simulink model "f_cd_reorder"  (R2018a)
settings: Solver=VariableStepAuto  StartTime=0.0  StopTime=200000  RelTol=1e-3
libraries: xbsIndex_r4 x1711, casper_library_misc x12, xps_library x2, simulink x1
(part 9 of 9)

== system f_cd_reorder/hmc_cd_reorder/reord/Subsystem/write_counter0 ==
  note: if there is a value missing we want to
      | increase by 1, if an enable we want to
      | increment by 2. If both then 3
  rst : Inport
  en : Inport  Port=2
  missing : Inport  Port=3
  AddSub2 : xbsIndex_r4/AddSub  mode=Addition  use_carryin=off  use_carryout=off  en=off  latency=0  precision=User Defined  arith_type=Unsigned  n_bits=n_bits_buffer  bin_pt=0  quantization=Truncate  overflow=Wrap  use_behavioral_HDL=on  hw_selection=Fabric  pipelined=off  dbl_ovrd=off  block_type=addsub
  Concat : xbsIndex_r4/Concat  num_inputs=2  dbl_ovrd=off  block_type=concat
  Constant : xbsIndex_r4/Constant  const=1  gui_display_data_type=Fixed-point  arith_type=Unsigned  n_bits=2  bin_pt=0  preci_type=Single  exp_width=8  frac_width=24  explicit_period=on  period=1  equ=P=C  opselect=C  inp2=PCIN>>17  opr=+  inp1=P  carry=CIN  dbl_ovrd=off  block_type=constant
  Constant1 : xbsIndex_r4/Constant  const=3  gui_display_data_type=Fixed-point  arith_type=Unsigned  n_bits=2  bin_pt=0  preci_type=Single  exp_width=8  frac_width=24  explicit_period=on  period=1  equ=P=C  opselect=C  inp2=PCIN>>17  opr=+  inp1=P  carry=CIN  dbl_ovrd=off  block_type=constant
  Constant2 : xbsIndex_r4/Constant  const=2  gui_display_data_type=Fixed-point  arith_type=Unsigned  n_bits=2  bin_pt=0  preci_type=Single  exp_width=8  frac_width=24  explicit_period=on  period=1  equ=P=C  opselect=C  inp2=PCIN>>17  opr=+  inp1=P  carry=CIN  dbl_ovrd=off  block_type=constant
  Constant3 : xbsIndex_r4/Constant  const=0  gui_display_data_type=Fixed-point  arith_type=Unsigned  n_bits=2  bin_pt=0  preci_type=Single  exp_width=8  frac_width=24  explicit_period=on  period=1  equ=P=C  opselect=C  inp2=PCIN>>17  opr=+  inp1=P  carry=CIN  dbl_ovrd=off  block_type=constant
  Delay13 : xbsIndex_r4/Delay  rst=off  infoeditControl=Selection of Reset will increase slice count due to use of real FFs and instead of SRLs  en=off  latency=1  reg_retiming=on  dbl_ovrd=off  block_type=delay
  Delay2 : xbsIndex_r4/Delay  rst=off  infoeditControl=Selection of Reset will increase slice count due to use of real FFs and instead of SRLs  en=off  latency=2  reg_retiming=on  dbl_ovrd=off  block_type=delay
  Delay3 : xbsIndex_r4/Delay  rst=off  infoeditControl=Selection of Reset will increase slice count due to use of real FFs and instead of SRLs  en=off  latency=2  reg_retiming=on  dbl_ovrd=off  block_type=delay
  Delay4 : xbsIndex_r4/Delay  rst=off  infoeditControl=Selection of Reset will increase slice count due to use of real FFs and instead of SRLs  en=off  latency=2  reg_retiming=on  dbl_ovrd=off  block_type=delay
  Gateway Out{,1..5} (6 alike) : xbsIndex_r4/Gateway Out  inherit_from_input=off  hdl_port=off  rows=1  columns=1  UseAsDAC=off  DACChannel='1'  interface=None  automatic_assignment=on  address_offset=hex2dec('00')  intf_name=''  intf_description=''  timing_constraint=None  locs_specified=off  LOCs={}  io_standard={}  block_type=gatewayout
  Logical8 : xbsIndex_r4/Logical  logical_function=OR  inputs=2  en=off  latency=1  precision=Full  arith_type=Unsigned  n_bits=16  bin_pt=0  align_bp=on  dbl_ovrd=off  block_type=logical
  Mux1 : xbsIndex_r4/Mux  inputs=4  en=off  latency=1  precision=Full  arith_type=Unsigned  n_bits=16  bin_pt=14  quantization=Truncate  overflow=Wrap  dbl_ovrd=off  block_type=mux
  Register : xbsIndex_r4/Register  init=0  rst=on  en=on  dbl_ovrd=off  block_type=register
  Scope : Scope  NumInputPorts=6
  count : Outport
  wires:
  en/1 -> Delay3/1
  AddSub2/1 -> Register/1, Gateway Out4/1
  rst/1 -> Delay4/1
  Delay13/1 -> Register/2
  missing/1 -> Delay2/1
  Logical8/1 -> Register/3
  Mux1/1 -> Gateway Out3/1, AddSub2/1
  Concat/1 -> Mux1/1
  Gateway Out/1 -> Scope/1
  Gateway Out1/1 -> Scope/2
  Gateway Out2/1 -> Scope/3
  Gateway Out3/1 -> Scope/4
  Gateway Out4/1 -> Scope/5
  Gateway Out5/1 -> Scope/6
  Constant3/1 -> Mux1/2
  Constant/1 -> Mux1/3
  Constant2/1 -> Mux1/4
  Constant1/1 -> Mux1/5
  Register/1 -> count/1, Gateway Out5/1, AddSub2/2
  Delay2/1 -> Logical8/1, Concat/2, Gateway Out1/1
  Delay3/1 -> Gateway Out2/1, Concat/1, Logical8/2
  Delay4/1 -> Delay13/1, Gateway Out/1

== system f_cd_reorder/hmc_cd_reorder/reord/Subsystem/write_counter1 ==
  note: if there is a value missing we want to
      | increase by 1, if an enable we want to
      | increment by 2. If both then 3
  rst : Inport
  en : Inport  Port=2
  missing : Inport  Port=3
  AddSub2 : xbsIndex_r4/AddSub  mode=Addition  use_carryin=off  use_carryout=off  en=off  latency=0  precision=User Defined  arith_type=Unsigned  n_bits=n_bits_buffer  bin_pt=0  quantization=Truncate  overflow=Wrap  use_behavioral_HDL=on  hw_selection=Fabric  pipelined=off  dbl_ovrd=off  block_type=addsub
  Concat : xbsIndex_r4/Concat  num_inputs=2  dbl_ovrd=off  block_type=concat
  Constant : xbsIndex_r4/Constant  const=1  gui_display_data_type=Fixed-point  arith_type=Unsigned  n_bits=2  bin_pt=0  preci_type=Single  exp_width=8  frac_width=24  explicit_period=on  period=1  equ=P=C  opselect=C  inp2=PCIN>>17  opr=+  inp1=P  carry=CIN  dbl_ovrd=off  block_type=constant
  Constant1 : xbsIndex_r4/Constant  const=3  gui_display_data_type=Fixed-point  arith_type=Unsigned  n_bits=2  bin_pt=0  preci_type=Single  exp_width=8  frac_width=24  explicit_period=on  period=1  equ=P=C  opselect=C  inp2=PCIN>>17  opr=+  inp1=P  carry=CIN  dbl_ovrd=off  block_type=constant
  Constant2 : xbsIndex_r4/Constant  const=2  gui_display_data_type=Fixed-point  arith_type=Unsigned  n_bits=2  bin_pt=0  preci_type=Single  exp_width=8  frac_width=24  explicit_period=on  period=1  equ=P=C  opselect=C  inp2=PCIN>>17  opr=+  inp1=P  carry=CIN  dbl_ovrd=off  block_type=constant
  Constant3 : xbsIndex_r4/Constant  const=0  gui_display_data_type=Fixed-point  arith_type=Unsigned  n_bits=2  bin_pt=0  preci_type=Single  exp_width=8  frac_width=24  explicit_period=on  period=1  equ=P=C  opselect=C  inp2=PCIN>>17  opr=+  inp1=P  carry=CIN  dbl_ovrd=off  block_type=constant
  Delay13 : xbsIndex_r4/Delay  rst=off  infoeditControl=Selection of Reset will increase slice count due to use of real FFs and instead of SRLs  en=off  latency=1  reg_retiming=on  dbl_ovrd=off  block_type=delay
  Delay2 : xbsIndex_r4/Delay  rst=off  infoeditControl=Selection of Reset will increase slice count due to use of real FFs and instead of SRLs  en=off  latency=2  reg_retiming=on  dbl_ovrd=off  block_type=delay
  Delay3 : xbsIndex_r4/Delay  rst=off  infoeditControl=Selection of Reset will increase slice count due to use of real FFs and instead of SRLs  en=off  latency=2  reg_retiming=on  dbl_ovrd=off  block_type=delay
  Delay4 : xbsIndex_r4/Delay  rst=off  infoeditControl=Selection of Reset will increase slice count due to use of real FFs and instead of SRLs  en=off  latency=2  reg_retiming=on  dbl_ovrd=off  block_type=delay
  Gateway Out{,1..5} (6 alike) : xbsIndex_r4/Gateway Out  inherit_from_input=off  hdl_port=off  rows=1  columns=1  UseAsDAC=off  DACChannel='1'  interface=None  automatic_assignment=on  address_offset=hex2dec('00')  intf_name=''  intf_description=''  timing_constraint=None  locs_specified=off  LOCs={}  io_standard={}  block_type=gatewayout
  Logical8 : xbsIndex_r4/Logical  logical_function=OR  inputs=2  en=off  latency=1  precision=Full  arith_type=Unsigned  n_bits=16  bin_pt=0  align_bp=on  dbl_ovrd=off  block_type=logical
  Mux1 : xbsIndex_r4/Mux  inputs=4  en=off  latency=1  precision=Full  arith_type=Unsigned  n_bits=16  bin_pt=14  quantization=Truncate  overflow=Wrap  dbl_ovrd=off  block_type=mux
  Register : xbsIndex_r4/Register  init=0  rst=on  en=on  dbl_ovrd=off  block_type=register
  Scope : Scope  NumInputPorts=6
  count : Outport
  wires:
  Delay4/1 -> Gateway Out/1, Delay13/1
  Delay3/1 -> Logical8/2, Concat/1, Gateway Out2/1
  Delay2/1 -> Gateway Out1/1, Concat/2, Logical8/1
  Register/1 -> AddSub2/2, Gateway Out5/1, count/1
  Constant1/1 -> Mux1/5
  Constant2/1 -> Mux1/4
  Constant/1 -> Mux1/3
  Constant3/1 -> Mux1/2
  Gateway Out5/1 -> Scope/6
  Gateway Out4/1 -> Scope/5
  Gateway Out3/1 -> Scope/4
  Gateway Out2/1 -> Scope/3
  Gateway Out1/1 -> Scope/2
  Gateway Out/1 -> Scope/1
  Concat/1 -> Mux1/1
  Mux1/1 -> AddSub2/1, Gateway Out3/1
  Logical8/1 -> Register/3
  missing/1 -> Delay2/1
  Delay13/1 -> Register/2
  rst/1 -> Delay4/1
  AddSub2/1 -> Gateway Out4/1, Register/1
  en/1 -> Delay3/1

== system f_cd_reorder/hmc_cd_reorder/reord/Subsystem/Subsystem1/Subsystem1 ==
  note: We mark when
      | we first receive
      | tags for this
      | quadrant in the buffer
  load : Inport
  tag : Inport  Port=2
  en : Inport  Port=3
  previous_quadrant : Inport  Port=4
  Constant1 : xbsIndex_r4/Constant  const=quadrant_index  gui_display_data_type=Fixed-point  arith_type=Unsigned  n_bits=2  bin_pt=0  preci_type=Single  exp_width=8  frac_width=24  explicit_period=on  period=1  equ=P=C  opselect=C  inp2=PCIN>>17  opr=+  inp1=P  carry=CIN  dbl_ovrd=off  block_type=constant
  Delay2 : xbsIndex_r4/Delay  rst=on  infoeditControl=Selection of Reset will increase slice count due to use of real FFs and instead of SRLs  en=on  latency=1  reg_retiming=on  dbl_ovrd=off  block_type=delay
  Gateway Out{,1..15} (16 alike) : xbsIndex_r4/Gateway Out  inherit_from_input=off  hdl_port=off  rows=1  columns=1  UseAsDAC=off  DACChannel='1'  interface=None  automatic_assignment=on  address_offset=hex2dec('00')  intf_name=''  intf_description=''  timing_constraint=None  locs_specified=off  LOCs={}  io_standard={}  block_type=gatewayout
  Logical1 : xbsIndex_r4/Logical  logical_function=AND  inputs=2  en=off  latency=0  precision=Full  arith_type=Unsigned  n_bits=16  bin_pt=0  align_bp=on  dbl_ovrd=off  block_type=logical
  Logical12 : xbsIndex_r4/Logical  logical_function=OR  inputs=2  en=off  latency=0  precision=Full  arith_type=Unsigned  n_bits=16  bin_pt=0  align_bp=on  dbl_ovrd=off  block_type=logical
  Logical5 : xbsIndex_r4/Logical  logical_function=AND  inputs=2  en=off  latency=0  precision=Full  arith_type=Unsigned  n_bits=16  bin_pt=0  align_bp=on  dbl_ovrd=off  block_type=logical
  Relational : xbsIndex_r4/Relational  mode=a=b  op_type=Bool  en=off  latency=0  dbl_ovrd=off  block_type=relational
  Scope : Scope  NumInputPorts=8
  Scope1 : Scope  NumInputPorts=4
  Scope2 : Scope  NumInputPorts=4
  edge_detect : casper_library_misc/edge_detect  edge=Rising  polarity=Active High  x_in=[0 0.08 0.08 0.16 0.16 0.24 0.24 0.32 0.32 0.4]  y_in="[-1 -1  1  1  1  1  1  1  1  1]"  x_out=[0.6 0.68 0.68 0.76 0.76 0.84 0.84 0.92 0.92 1]  y_out="[-1 -1  1  1 -1 -1 -1 -1 -1 -1]"
  quadrant_offset_count : xbsIndex_r4/Counter  cnt_type=Free Running  cnt_to=Inf  operation=Up  start_count=0  cnt_by_val=1  arith_type=Unsigned  n_bits=n_bits_buffer-10  bin_pt=0  load_pin=off  rst=on  en=on  explicit_period=on  period=1  use_behavioral_HDL=off  implementation=Fabric  dbl_ovrd=off  block_type=counter
  quadrant_offset : Outport
  tags_received : Outport  Port=2
  wires:
  Logical5/1 -> Delay2/3, Delay2/1, Gateway Out4/1
  en/1 -> Gateway Out3/1, Logical5/2
  Delay2/1 -> Logical1/2, tags_received/1, Gateway Out6/1, Gateway Out12/1
  Constant1/1 -> Relational/2
  load/1 -> Gateway Out9/1, Gateway Out8/1, quadrant_offset_count/1, Logical12/1, Gateway Out/1
  quadrant_offset_count/1 -> Gateway Out11/1, quadrant_offset/1
  tag/1 -> Gateway Out2/1, Relational/1
  Relational/1 -> Logical5/1
  Logical1/1 -> Gateway Out10/1, quadrant_offset_count/2, Gateway Out13/1, Gateway Out7/1, Logical12/2
  Logical12/1 -> Delay2/2, Gateway Out5/1
  previous_quadrant/1 -> Gateway Out14/1, edge_detect/1, Gateway Out1/1
  Gateway Out2/1 -> Scope/3
  Gateway Out3/1 -> Scope/4
  Gateway Out1/1 -> Scope/2
  Gateway Out/1 -> Scope/1
  Gateway Out4/1 -> Scope/5
  Gateway Out5/1 -> Scope/6
  Gateway Out6/1 -> Scope/7
  Gateway Out7/1 -> Scope/8
  Gateway Out8/1 -> Scope1/1
  Gateway Out9/1 -> Scope1/2
  Gateway Out10/1 -> Scope1/3
  Gateway Out11/1 -> Scope1/4
  Gateway Out13/1 -> Scope2/4
  Gateway Out12/1 -> Scope2/3
  Gateway Out15/1 -> Scope2/2
  Gateway Out14/1 -> Scope2/1
  edge_detect/1 -> Logical1/1, Gateway Out15/1

== system f_cd_reorder/hmc_cd_reorder/reord/Subsystem/Subsystem1/Subsystem2 ==
  note: We mark when
      | we first receive
      | tags for this
      | quadrant in the buffer
  load : Inport
  tag : Inport  Port=2
  en : Inport  Port=3
  previous_quadrant : Inport  Port=4
  Constant1 : xbsIndex_r4/Constant  const=quadrant_index  gui_display_data_type=Fixed-point  arith_type=Unsigned  n_bits=2  bin_pt=0  preci_type=Single  exp_width=8  frac_width=24  explicit_period=on  period=1  equ=P=C  opselect=C  inp2=PCIN>>17  opr=+  inp1=P  carry=CIN  dbl_ovrd=off  block_type=constant
  Delay2 : xbsIndex_r4/Delay  rst=on  infoeditControl=Selection of Reset will increase slice count due to use of real FFs and instead of SRLs  en=on  latency=1  reg_retiming=on  dbl_ovrd=off  block_type=delay
  Gateway Out{,1..15} (16 alike) : xbsIndex_r4/Gateway Out  inherit_from_input=off  hdl_port=off  rows=1  columns=1  UseAsDAC=off  DACChannel='1'  interface=None  automatic_assignment=on  address_offset=hex2dec('00')  intf_name=''  intf_description=''  timing_constraint=None  locs_specified=off  LOCs={}  io_standard={}  block_type=gatewayout
  Logical1 : xbsIndex_r4/Logical  logical_function=AND  inputs=2  en=off  latency=0  precision=Full  arith_type=Unsigned  n_bits=16  bin_pt=0  align_bp=on  dbl_ovrd=off  block_type=logical
  Logical12 : xbsIndex_r4/Logical  logical_function=OR  inputs=2  en=off  latency=0  precision=Full  arith_type=Unsigned  n_bits=16  bin_pt=0  align_bp=on  dbl_ovrd=off  block_type=logical
  Logical5 : xbsIndex_r4/Logical  logical_function=AND  inputs=2  en=off  latency=0  precision=Full  arith_type=Unsigned  n_bits=16  bin_pt=0  align_bp=on  dbl_ovrd=off  block_type=logical
  Relational : xbsIndex_r4/Relational  mode=a=b  op_type=Bool  en=off  latency=0  dbl_ovrd=off  block_type=relational
  Scope : Scope  NumInputPorts=8
  Scope1 : Scope  NumInputPorts=4
  Scope2 : Scope  NumInputPorts=4
  edge_detect : casper_library_misc/edge_detect  edge=Rising  polarity=Active High  x_in=[0 0.08 0.08 0.16 0.16 0.24 0.24 0.32 0.32 0.4]  y_in="[-1 -1  1  1  1  1  1  1  1  1]"  x_out=[0.6 0.68 0.68 0.76 0.76 0.84 0.84 0.92 0.92 1]  y_out="[-1 -1  1  1 -1 -1 -1 -1 -1 -1]"
  quadrant_offset_count : xbsIndex_r4/Counter  cnt_type=Free Running  cnt_to=Inf  operation=Up  start_count=0  cnt_by_val=1  arith_type=Unsigned  n_bits=n_bits_buffer-10  bin_pt=0  load_pin=off  rst=on  en=on  explicit_period=on  period=1  use_behavioral_HDL=off  implementation=Fabric  dbl_ovrd=off  block_type=counter
  quadrant_offset : Outport
  tags_received : Outport  Port=2
  wires:
  edge_detect/1 -> Gateway Out15/1, Logical1/1
  Gateway Out14/1 -> Scope2/1
  Gateway Out15/1 -> Scope2/2
  Gateway Out12/1 -> Scope2/3
  Gateway Out13/1 -> Scope2/4
  Gateway Out11/1 -> Scope1/4
  Gateway Out10/1 -> Scope1/3
  Gateway Out9/1 -> Scope1/2
  Gateway Out8/1 -> Scope1/1
  Gateway Out7/1 -> Scope/8
  Gateway Out6/1 -> Scope/7
  Gateway Out5/1 -> Scope/6
  Gateway Out4/1 -> Scope/5
  Gateway Out/1 -> Scope/1
  Gateway Out1/1 -> Scope/2
  Gateway Out3/1 -> Scope/4
  Gateway Out2/1 -> Scope/3
  previous_quadrant/1 -> Gateway Out1/1, edge_detect/1, Gateway Out14/1
  Logical12/1 -> Gateway Out5/1, Delay2/2
  Logical1/1 -> Logical12/2, Gateway Out7/1, Gateway Out13/1, quadrant_offset_count/2, Gateway Out10/1
  Relational/1 -> Logical5/1
  tag/1 -> Relational/1, Gateway Out2/1
  quadrant_offset_count/1 -> quadrant_offset/1, Gateway Out11/1
  load/1 -> Gateway Out/1, Logical12/1, quadrant_offset_count/1, Gateway Out8/1, Gateway Out9/1
  Constant1/1 -> Relational/2
  Delay2/1 -> Gateway Out12/1, Gateway Out6/1, tags_received/1, Logical1/2
  en/1 -> Logical5/2, Gateway Out3/1
  Logical5/1 -> Gateway Out4/1, Delay2/1, Delay2/3

== system f_cd_reorder/hmc_cd_reorder/reord/Subsystem/Subsystem1/Subsystem3 ==
  note: We mark when
      | we first receive
      | tags for this
      | quadrant in the buffer
  load : Inport
  tag : Inport  Port=2
  en : Inport  Port=3
  previous_quadrant : Inport  Port=4
  Constant1 : xbsIndex_r4/Constant  const=quadrant_index  gui_display_data_type=Fixed-point  arith_type=Unsigned  n_bits=2  bin_pt=0  preci_type=Single  exp_width=8  frac_width=24  explicit_period=on  period=1  equ=P=C  opselect=C  inp2=PCIN>>17  opr=+  inp1=P  carry=CIN  dbl_ovrd=off  block_type=constant
  Delay2 : xbsIndex_r4/Delay  rst=on  infoeditControl=Selection of Reset will increase slice count due to use of real FFs and instead of SRLs  en=on  latency=1  reg_retiming=on  dbl_ovrd=off  block_type=delay
  Gateway Out{,1..15} (16 alike) : xbsIndex_r4/Gateway Out  inherit_from_input=off  hdl_port=off  rows=1  columns=1  UseAsDAC=off  DACChannel='1'  interface=None  automatic_assignment=on  address_offset=hex2dec('00')  intf_name=''  intf_description=''  timing_constraint=None  locs_specified=off  LOCs={}  io_standard={}  block_type=gatewayout
  Logical1 : xbsIndex_r4/Logical  logical_function=AND  inputs=2  en=off  latency=0  precision=Full  arith_type=Unsigned  n_bits=16  bin_pt=0  align_bp=on  dbl_ovrd=off  block_type=logical
  Logical12 : xbsIndex_r4/Logical  logical_function=OR  inputs=2  en=off  latency=0  precision=Full  arith_type=Unsigned  n_bits=16  bin_pt=0  align_bp=on  dbl_ovrd=off  block_type=logical
  Logical5 : xbsIndex_r4/Logical  logical_function=AND  inputs=2  en=off  latency=0  precision=Full  arith_type=Unsigned  n_bits=16  bin_pt=0  align_bp=on  dbl_ovrd=off  block_type=logical
  Relational : xbsIndex_r4/Relational  mode=a=b  op_type=Bool  en=off  latency=0  dbl_ovrd=off  block_type=relational
  Scope : Scope  NumInputPorts=8
  Scope1 : Scope  NumInputPorts=4
  Scope2 : Scope  NumInputPorts=4
  edge_detect : casper_library_misc/edge_detect  edge=Rising  polarity=Active High  x_in=[0 0.08 0.08 0.16 0.16 0.24 0.24 0.32 0.32 0.4]  y_in="[-1 -1  1  1  1  1  1  1  1  1]"  x_out=[0.6 0.68 0.68 0.76 0.76 0.84 0.84 0.92 0.92 1]  y_out="[-1 -1  1  1 -1 -1 -1 -1 -1 -1]"
  quadrant_offset_count : xbsIndex_r4/Counter  cnt_type=Free Running  cnt_to=Inf  operation=Up  start_count=0  cnt_by_val=1  arith_type=Unsigned  n_bits=n_bits_buffer-10  bin_pt=0  load_pin=off  rst=on  en=on  explicit_period=on  period=1  use_behavioral_HDL=off  implementation=Fabric  dbl_ovrd=off  block_type=counter
  quadrant_offset : Outport
  tags_received : Outport  Port=2
  wires:
  Logical5/1 -> Delay2/3, Delay2/1, Gateway Out4/1
  en/1 -> Gateway Out3/1, Logical5/2
  Delay2/1 -> Logical1/2, tags_received/1, Gateway Out6/1, Gateway Out12/1
  Constant1/1 -> Relational/2
  load/1 -> Gateway Out9/1, Gateway Out8/1, quadrant_offset_count/1, Logical12/1, Gateway Out/1
  quadrant_offset_count/1 -> Gateway Out11/1, quadrant_offset/1
  tag/1 -> Gateway Out2/1, Relational/1
  Relational/1 -> Logical5/1
  Logical1/1 -> Gateway Out10/1, quadrant_offset_count/2, Gateway Out13/1, Gateway Out7/1, Logical12/2
  Logical12/1 -> Delay2/2, Gateway Out5/1
  previous_quadrant/1 -> Gateway Out14/1, edge_detect/1, Gateway Out1/1
  Gateway Out2/1 -> Scope/3
  Gateway Out3/1 -> Scope/4
  Gateway Out1/1 -> Scope/2
  Gateway Out/1 -> Scope/1
  Gateway Out4/1 -> Scope/5
  Gateway Out5/1 -> Scope/6
  Gateway Out6/1 -> Scope/7
  Gateway Out7/1 -> Scope/8
  Gateway Out8/1 -> Scope1/1
  Gateway Out9/1 -> Scope1/2
  Gateway Out10/1 -> Scope1/3
  Gateway Out11/1 -> Scope1/4
  Gateway Out13/1 -> Scope2/4
  Gateway Out12/1 -> Scope2/3
  Gateway Out15/1 -> Scope2/2
  Gateway Out14/1 -> Scope2/1
  edge_detect/1 -> Logical1/1, Gateway Out15/1

== system f_cd_reorder/hmc_cd_reorder/reord/Subsystem/Subsystem1/Subsystem4 ==
  note: We mark when
      | we first receive
      | tags for this
      | quadrant in the buffer
  load : Inport
  tag : Inport  Port=2
  en : Inport  Port=3
  previous_quadrant : Inport  Port=4
  Constant1 : xbsIndex_r4/Constant  const=quadrant_index  gui_display_data_type=Fixed-point  arith_type=Unsigned  n_bits=2  bin_pt=0  preci_type=Single  exp_width=8  frac_width=24  explicit_period=on  period=1  equ=P=C  opselect=C  inp2=PCIN>>17  opr=+  inp1=P  carry=CIN  dbl_ovrd=off  block_type=constant
  Delay2 : xbsIndex_r4/Delay  rst=on  infoeditControl=Selection of Reset will increase slice count due to use of real FFs and instead of SRLs  en=on  latency=1  reg_retiming=on  dbl_ovrd=off  block_type=delay
  Gateway Out{,1..15} (16 alike) : xbsIndex_r4/Gateway Out  inherit_from_input=off  hdl_port=off  rows=1  columns=1  UseAsDAC=off  DACChannel='1'  interface=None  automatic_assignment=on  address_offset=hex2dec('00')  intf_name=''  intf_description=''  timing_constraint=None  locs_specified=off  LOCs={}  io_standard={}  block_type=gatewayout
  Logical1 : xbsIndex_r4/Logical  logical_function=AND  inputs=2  en=off  latency=0  precision=Full  arith_type=Unsigned  n_bits=16  bin_pt=0  align_bp=on  dbl_ovrd=off  block_type=logical
  Logical12 : xbsIndex_r4/Logical  logical_function=OR  inputs=2  en=off  latency=0  precision=Full  arith_type=Unsigned  n_bits=16  bin_pt=0  align_bp=on  dbl_ovrd=off  block_type=logical
  Logical5 : xbsIndex_r4/Logical  logical_function=AND  inputs=2  en=off  latency=0  precision=Full  arith_type=Unsigned  n_bits=16  bin_pt=0  align_bp=on  dbl_ovrd=off  block_type=logical
  Relational : xbsIndex_r4/Relational  mode=a=b  op_type=Bool  en=off  latency=0  dbl_ovrd=off  block_type=relational
  Scope : Scope  NumInputPorts=8
  Scope1 : Scope  NumInputPorts=4
  Scope2 : Scope  NumInputPorts=4
  edge_detect : casper_library_misc/edge_detect  edge=Rising  polarity=Active High  x_in=[0 0.08 0.08 0.16 0.16 0.24 0.24 0.32 0.32 0.4]  y_in="[-1 -1  1  1  1  1  1  1  1  1]"  x_out=[0.6 0.68 0.68 0.76 0.76 0.84 0.84 0.92 0.92 1]  y_out="[-1 -1  1  1 -1 -1 -1 -1 -1 -1]"
  quadrant_offset_count : xbsIndex_r4/Counter  cnt_type=Free Running  cnt_to=Inf  operation=Up  start_count=0  cnt_by_val=1  arith_type=Unsigned  n_bits=n_bits_buffer-10  bin_pt=0  load_pin=off  rst=on  en=on  explicit_period=on  period=1  use_behavioral_HDL=off  implementation=Fabric  dbl_ovrd=off  block_type=counter
  quadrant_offset : Outport
  tags_received : Outport  Port=2
  wires:
  edge_detect/1 -> Gateway Out15/1, Logical1/1
  Gateway Out14/1 -> Scope2/1
  Gateway Out15/1 -> Scope2/2
  Gateway Out12/1 -> Scope2/3
  Gateway Out13/1 -> Scope2/4
  Gateway Out11/1 -> Scope1/4
  Gateway Out10/1 -> Scope1/3
  Gateway Out9/1 -> Scope1/2
  Gateway Out8/1 -> Scope1/1
  Gateway Out7/1 -> Scope/8
  Gateway Out6/1 -> Scope/7
  Gateway Out5/1 -> Scope/6
  Gateway Out4/1 -> Scope/5
  Gateway Out/1 -> Scope/1
  Gateway Out1/1 -> Scope/2
  Gateway Out3/1 -> Scope/4
  Gateway Out2/1 -> Scope/3
  previous_quadrant/1 -> Gateway Out1/1, edge_detect/1, Gateway Out14/1
  Logical12/1 -> Gateway Out5/1, Delay2/2
  Logical1/1 -> Logical12/2, Gateway Out7/1, Gateway Out13/1, quadrant_offset_count/2, Gateway Out10/1
  Relational/1 -> Logical5/1
  tag/1 -> Relational/1, Gateway Out2/1
  quadrant_offset_count/1 -> quadrant_offset/1, Gateway Out11/1
  load/1 -> Gateway Out/1, Logical12/1, quadrant_offset_count/1, Gateway Out8/1, Gateway Out9/1
  Constant1/1 -> Relational/2
  Delay2/1 -> Gateway Out12/1, Gateway Out6/1, tags_received/1, Logical1/2
  en/1 -> Logical5/2, Gateway Out3/1
  Logical5/1 -> Gateway Out4/1, Delay2/1, Delay2/3

== system f_cd_reorder/hmc_cd_reorder/reord/Subsystem/Subsystem2/Subsystem1 ==
  note: We mark when
      | we first receive
      | tags for this
      | quadrant in the buffer
  load : Inport
  tag : Inport  Port=2
  en : Inport  Port=3
  previous_quadrant : Inport  Port=4
  Constant1 : xbsIndex_r4/Constant  const=quadrant_index  gui_display_data_type=Fixed-point  arith_type=Unsigned  n_bits=2  bin_pt=0  preci_type=Single  exp_width=8  frac_width=24  explicit_period=on  period=1  equ=P=C  opselect=C  inp2=PCIN>>17  opr=+  inp1=P  carry=CIN  dbl_ovrd=off  block_type=constant
  Delay2 : xbsIndex_r4/Delay  rst=on  infoeditControl=Selection of Reset will increase slice count due to use of real FFs and instead of SRLs  en=on  latency=1  reg_retiming=on  dbl_ovrd=off  block_type=delay
  Gateway Out{,1..15} (16 alike) : xbsIndex_r4/Gateway Out  inherit_from_input=off  hdl_port=off  rows=1  columns=1  UseAsDAC=off  DACChannel='1'  interface=None  automatic_assignment=on  address_offset=hex2dec('00')  intf_name=''  intf_description=''  timing_constraint=None  locs_specified=off  LOCs={}  io_standard={}  block_type=gatewayout
  Logical1 : xbsIndex_r4/Logical  logical_function=AND  inputs=2  en=off  latency=0  precision=Full  arith_type=Unsigned  n_bits=16  bin_pt=0  align_bp=on  dbl_ovrd=off  block_type=logical
  Logical12 : xbsIndex_r4/Logical  logical_function=OR  inputs=2  en=off  latency=0  precision=Full  arith_type=Unsigned  n_bits=16  bin_pt=0  align_bp=on  dbl_ovrd=off  block_type=logical
  Logical5 : xbsIndex_r4/Logical  logical_function=AND  inputs=2  en=off  latency=0  precision=Full  arith_type=Unsigned  n_bits=16  bin_pt=0  align_bp=on  dbl_ovrd=off  block_type=logical
  Relational : xbsIndex_r4/Relational  mode=a=b  op_type=Bool  en=off  latency=0  dbl_ovrd=off  block_type=relational
  Scope : Scope  NumInputPorts=8
  Scope1 : Scope  NumInputPorts=4
  Scope2 : Scope  NumInputPorts=4
  edge_detect : casper_library_misc/edge_detect  edge=Rising  polarity=Active High  x_in=[0 0.08 0.08 0.16 0.16 0.24 0.24 0.32 0.32 0.4]  y_in="[-1 -1  1  1  1  1  1  1  1  1]"  x_out=[0.6 0.68 0.68 0.76 0.76 0.84 0.84 0.92 0.92 1]  y_out="[-1 -1  1  1 -1 -1 -1 -1 -1 -1]"
  quadrant_offset_count : xbsIndex_r4/Counter  cnt_type=Free Running  cnt_to=Inf  operation=Up  start_count=0  cnt_by_val=1  arith_type=Unsigned  n_bits=n_bits_buffer-10  bin_pt=0  load_pin=off  rst=on  en=on  explicit_period=on  period=1  use_behavioral_HDL=off  implementation=Fabric  dbl_ovrd=off  block_type=counter
  quadrant_offset : Outport
  tags_received : Outport  Port=2
  wires:
  edge_detect/1 -> Gateway Out15/1, Logical1/1
  Gateway Out14/1 -> Scope2/1
  Gateway Out15/1 -> Scope2/2
  Gateway Out12/1 -> Scope2/3
  Gateway Out13/1 -> Scope2/4
  Gateway Out11/1 -> Scope1/4
  Gateway Out10/1 -> Scope1/3
  Gateway Out9/1 -> Scope1/2
  Gateway Out8/1 -> Scope1/1
  Gateway Out7/1 -> Scope/8
  Gateway Out6/1 -> Scope/7
  Gateway Out5/1 -> Scope/6
  Gateway Out4/1 -> Scope/5
  Gateway Out/1 -> Scope/1
  Gateway Out1/1 -> Scope/2
  Gateway Out3/1 -> Scope/4
  Gateway Out2/1 -> Scope/3
  previous_quadrant/1 -> Gateway Out1/1, edge_detect/1, Gateway Out14/1
  Logical12/1 -> Gateway Out5/1, Delay2/2
  Logical1/1 -> Logical12/2, Gateway Out7/1, Gateway Out13/1, quadrant_offset_count/2, Gateway Out10/1
  Relational/1 -> Logical5/1
  tag/1 -> Relational/1, Gateway Out2/1
  quadrant_offset_count/1 -> quadrant_offset/1, Gateway Out11/1
  load/1 -> Gateway Out/1, Logical12/1, quadrant_offset_count/1, Gateway Out8/1, Gateway Out9/1
  Constant1/1 -> Relational/2
  Delay2/1 -> Gateway Out12/1, Gateway Out6/1, tags_received/1, Logical1/2
  en/1 -> Logical5/2, Gateway Out3/1
  Logical5/1 -> Gateway Out4/1, Delay2/1, Delay2/3

== system f_cd_reorder/hmc_cd_reorder/reord/Subsystem/Subsystem2/Subsystem2 ==
  note: We mark when
      | we first receive
      | tags for this
      | quadrant in the buffer
  load : Inport
  tag : Inport  Port=2
  en : Inport  Port=3
  previous_quadrant : Inport  Port=4
  Constant1 : xbsIndex_r4/Constant  const=quadrant_index  gui_display_data_type=Fixed-point  arith_type=Unsigned  n_bits=2  bin_pt=0  preci_type=Single  exp_width=8  frac_width=24  explicit_period=on  period=1  equ=P=C  opselect=C  inp2=PCIN>>17  opr=+  inp1=P  carry=CIN  dbl_ovrd=off  block_type=constant
  Delay2 : xbsIndex_r4/Delay  rst=on  infoeditControl=Selection of Reset will increase slice count due to use of real FFs and instead of SRLs  en=on  latency=1  reg_retiming=on  dbl_ovrd=off  block_type=delay
  Gateway Out{,1..15} (16 alike) : xbsIndex_r4/Gateway Out  inherit_from_input=off  hdl_port=off  rows=1  columns=1  UseAsDAC=off  DACChannel='1'  interface=None  automatic_assignment=on  address_offset=hex2dec('00')  intf_name=''  intf_description=''  timing_constraint=None  locs_specified=off  LOCs={}  io_standard={}  block_type=gatewayout
  Logical1 : xbsIndex_r4/Logical  logical_function=AND  inputs=2  en=off  latency=0  precision=Full  arith_type=Unsigned  n_bits=16  bin_pt=0  align_bp=on  dbl_ovrd=off  block_type=logical
  Logical12 : xbsIndex_r4/Logical  logical_function=OR  inputs=2  en=off  latency=0  precision=Full  arith_type=Unsigned  n_bits=16  bin_pt=0  align_bp=on  dbl_ovrd=off  block_type=logical
  Logical5 : xbsIndex_r4/Logical  logical_function=AND  inputs=2  en=off  latency=0  precision=Full  arith_type=Unsigned  n_bits=16  bin_pt=0  align_bp=on  dbl_ovrd=off  block_type=logical
  Relational : xbsIndex_r4/Relational  mode=a=b  op_type=Bool  en=off  latency=0  dbl_ovrd=off  block_type=relational
  Scope : Scope  NumInputPorts=8
  Scope1 : Scope  NumInputPorts=4
  Scope2 : Scope  NumInputPorts=4
  edge_detect : casper_library_misc/edge_detect  edge=Rising  polarity=Active High  x_in=[0 0.08 0.08 0.16 0.16 0.24 0.24 0.32 0.32 0.4]  y_in="[-1 -1  1  1  1  1  1  1  1  1]"  x_out=[0.6 0.68 0.68 0.76 0.76 0.84 0.84 0.92 0.92 1]  y_out="[-1 -1  1  1 -1 -1 -1 -1 -1 -1]"
  quadrant_offset_count : xbsIndex_r4/Counter  cnt_type=Free Running  cnt_to=Inf  operation=Up  start_count=0  cnt_by_val=1  arith_type=Unsigned  n_bits=n_bits_buffer-10  bin_pt=0  load_pin=off  rst=on  en=on  explicit_period=on  period=1  use_behavioral_HDL=off  implementation=Fabric  dbl_ovrd=off  block_type=counter
  quadrant_offset : Outport
  tags_received : Outport  Port=2
  wires:
  Logical5/1 -> Delay2/3, Delay2/1, Gateway Out4/1
  en/1 -> Gateway Out3/1, Logical5/2
  Delay2/1 -> Logical1/2, tags_received/1, Gateway Out6/1, Gateway Out12/1
  Constant1/1 -> Relational/2
  load/1 -> Gateway Out9/1, Gateway Out8/1, quadrant_offset_count/1, Logical12/1, Gateway Out/1
  quadrant_offset_count/1 -> Gateway Out11/1, quadrant_offset/1
  tag/1 -> Gateway Out2/1, Relational/1
  Relational/1 -> Logical5/1
  Logical1/1 -> Gateway Out10/1, quadrant_offset_count/2, Gateway Out13/1, Gateway Out7/1, Logical12/2
  Logical12/1 -> Delay2/2, Gateway Out5/1
  previous_quadrant/1 -> Gateway Out14/1, edge_detect/1, Gateway Out1/1
  Gateway Out2/1 -> Scope/3
  Gateway Out3/1 -> Scope/4
  Gateway Out1/1 -> Scope/2
  Gateway Out/1 -> Scope/1
  Gateway Out4/1 -> Scope/5
  Gateway Out5/1 -> Scope/6
  Gateway Out6/1 -> Scope/7
  Gateway Out7/1 -> Scope/8
  Gateway Out8/1 -> Scope1/1
  Gateway Out9/1 -> Scope1/2
  Gateway Out10/1 -> Scope1/3
  Gateway Out11/1 -> Scope1/4
  Gateway Out13/1 -> Scope2/4
  Gateway Out12/1 -> Scope2/3
  Gateway Out15/1 -> Scope2/2
  Gateway Out14/1 -> Scope2/1
  edge_detect/1 -> Logical1/1, Gateway Out15/1

== system f_cd_reorder/hmc_cd_reorder/reord/Subsystem/Subsystem2/Subsystem3 ==
  note: We mark when
      | we first receive
      | tags for this
      | quadrant in the buffer
  load : Inport
  tag : Inport  Port=2
  en : Inport  Port=3
  previous_quadrant : Inport  Port=4
  Constant1 : xbsIndex_r4/Constant  const=quadrant_index  gui_display_data_type=Fixed-point  arith_type=Unsigned  n_bits=2  bin_pt=0  preci_type=Single  exp_width=8  frac_width=24  explicit_period=on  period=1  equ=P=C  opselect=C  inp2=PCIN>>17  opr=+  inp1=P  carry=CIN  dbl_ovrd=off  block_type=constant
  Delay2 : xbsIndex_r4/Delay  rst=on  infoeditControl=Selection of Reset will increase slice count due to use of real FFs and instead of SRLs  en=on  latency=1  reg_retiming=on  dbl_ovrd=off  block_type=delay
  Gateway Out{,1..15} (16 alike) : xbsIndex_r4/Gateway Out  inherit_from_input=off  hdl_port=off  rows=1  columns=1  UseAsDAC=off  DACChannel='1'  interface=None  automatic_assignment=on  address_offset=hex2dec('00')  intf_name=''  intf_description=''  timing_constraint=None  locs_specified=off  LOCs={}  io_standard={}  block_type=gatewayout
  Logical1 : xbsIndex_r4/Logical  logical_function=AND  inputs=2  en=off  latency=0  precision=Full  arith_type=Unsigned  n_bits=16  bin_pt=0  align_bp=on  dbl_ovrd=off  block_type=logical
  Logical12 : xbsIndex_r4/Logical  logical_function=OR  inputs=2  en=off  latency=0  precision=Full  arith_type=Unsigned  n_bits=16  bin_pt=0  align_bp=on  dbl_ovrd=off  block_type=logical
  Logical5 : xbsIndex_r4/Logical  logical_function=AND  inputs=2  en=off  latency=0  precision=Full  arith_type=Unsigned  n_bits=16  bin_pt=0  align_bp=on  dbl_ovrd=off  block_type=logical
  Relational : xbsIndex_r4/Relational  mode=a=b  op_type=Bool  en=off  latency=0  dbl_ovrd=off  block_type=relational
  Scope : Scope  NumInputPorts=8
  Scope1 : Scope  NumInputPorts=4
  Scope2 : Scope  NumInputPorts=4
  edge_detect : casper_library_misc/edge_detect  edge=Rising  polarity=Active High  x_in=[0 0.08 0.08 0.16 0.16 0.24 0.24 0.32 0.32 0.4]  y_in="[-1 -1  1  1  1  1  1  1  1  1]"  x_out=[0.6 0.68 0.68 0.76 0.76 0.84 0.84 0.92 0.92 1]  y_out="[-1 -1  1  1 -1 -1 -1 -1 -1 -1]"
  quadrant_offset_count : xbsIndex_r4/Counter  cnt_type=Free Running  cnt_to=Inf  operation=Up  start_count=0  cnt_by_val=1  arith_type=Unsigned  n_bits=n_bits_buffer-10  bin_pt=0  load_pin=off  rst=on  en=on  explicit_period=on  period=1  use_behavioral_HDL=off  implementation=Fabric  dbl_ovrd=off  block_type=counter
  quadrant_offset : Outport
  tags_received : Outport  Port=2
  wires:
  edge_detect/1 -> Gateway Out15/1, Logical1/1
  Gateway Out14/1 -> Scope2/1
  Gateway Out15/1 -> Scope2/2
  Gateway Out12/1 -> Scope2/3
  Gateway Out13/1 -> Scope2/4
  Gateway Out11/1 -> Scope1/4
  Gateway Out10/1 -> Scope1/3
  Gateway Out9/1 -> Scope1/2
  Gateway Out8/1 -> Scope1/1
  Gateway Out7/1 -> Scope/8
  Gateway Out6/1 -> Scope/7
  Gateway Out5/1 -> Scope/6
  Gateway Out4/1 -> Scope/5
  Gateway Out/1 -> Scope/1
  Gateway Out1/1 -> Scope/2
  Gateway Out3/1 -> Scope/4
  Gateway Out2/1 -> Scope/3
  previous_quadrant/1 -> Gateway Out1/1, edge_detect/1, Gateway Out14/1
  Logical12/1 -> Gateway Out5/1, Delay2/2
  Logical1/1 -> Logical12/2, Gateway Out7/1, Gateway Out13/1, quadrant_offset_count/2, Gateway Out10/1
  Relational/1 -> Logical5/1
  tag/1 -> Relational/1, Gateway Out2/1
  quadrant_offset_count/1 -> quadrant_offset/1, Gateway Out11/1
  load/1 -> Gateway Out/1, Logical12/1, quadrant_offset_count/1, Gateway Out8/1, Gateway Out9/1
  Constant1/1 -> Relational/2
  Delay2/1 -> Gateway Out12/1, Gateway Out6/1, tags_received/1, Logical1/2
  en/1 -> Logical5/2, Gateway Out3/1
  Logical5/1 -> Gateway Out4/1, Delay2/1, Delay2/3

== system f_cd_reorder/hmc_cd_reorder/reord/Subsystem/Subsystem2/Subsystem4 ==
  note: We mark when
      | we first receive
      | tags for this
      | quadrant in the buffer
  load : Inport
  tag : Inport  Port=2
  en : Inport  Port=3
  previous_quadrant : Inport  Port=4
  Constant1 : xbsIndex_r4/Constant  const=quadrant_index  gui_display_data_type=Fixed-point  arith_type=Unsigned  n_bits=2  bin_pt=0  preci_type=Single  exp_width=8  frac_width=24  explicit_period=on  period=1  equ=P=C  opselect=C  inp2=PCIN>>17  opr=+  inp1=P  carry=CIN  dbl_ovrd=off  block_type=constant
  Delay2 : xbsIndex_r4/Delay  rst=on  infoeditControl=Selection of Reset will increase slice count due to use of real FFs and instead of SRLs  en=on  latency=1  reg_retiming=on  dbl_ovrd=off  block_type=delay
  Gateway Out{,1..15} (16 alike) : xbsIndex_r4/Gateway Out  inherit_from_input=off  hdl_port=off  rows=1  columns=1  UseAsDAC=off  DACChannel='1'  interface=None  automatic_assignment=on  address_offset=hex2dec('00')  intf_name=''  intf_description=''  timing_constraint=None  locs_specified=off  LOCs={}  io_standard={}  block_type=gatewayout
  Logical1 : xbsIndex_r4/Logical  logical_function=AND  inputs=2  en=off  latency=0  precision=Full  arith_type=Unsigned  n_bits=16  bin_pt=0  align_bp=on  dbl_ovrd=off  block_type=logical
  Logical12 : xbsIndex_r4/Logical  logical_function=OR  inputs=2  en=off  latency=0  precision=Full  arith_type=Unsigned  n_bits=16  bin_pt=0  align_bp=on  dbl_ovrd=off  block_type=logical
  Logical5 : xbsIndex_r4/Logical  logical_function=AND  inputs=2  en=off  latency=0  precision=Full  arith_type=Unsigned  n_bits=16  bin_pt=0  align_bp=on  dbl_ovrd=off  block_type=logical
  Relational : xbsIndex_r4/Relational  mode=a=b  op_type=Bool  en=off  latency=0  dbl_ovrd=off  block_type=relational
  Scope : Scope  NumInputPorts=8
  Scope1 : Scope  NumInputPorts=4
  Scope2 : Scope  NumInputPorts=4
  edge_detect : casper_library_misc/edge_detect  edge=Rising  polarity=Active High  x_in=[0 0.08 0.08 0.16 0.16 0.24 0.24 0.32 0.32 0.4]  y_in="[-1 -1  1  1  1  1  1  1  1  1]"  x_out=[0.6 0.68 0.68 0.76 0.76 0.84 0.84 0.92 0.92 1]  y_out="[-1 -1  1  1 -1 -1 -1 -1 -1 -1]"
  quadrant_offset_count : xbsIndex_r4/Counter  cnt_type=Free Running  cnt_to=Inf  operation=Up  start_count=0  cnt_by_val=1  arith_type=Unsigned  n_bits=n_bits_buffer-10  bin_pt=0  load_pin=off  rst=on  en=on  explicit_period=on  period=1  use_behavioral_HDL=off  implementation=Fabric  dbl_ovrd=off  block_type=counter
  quadrant_offset : Outport
  tags_received : Outport  Port=2
  wires:
  Logical5/1 -> Delay2/3, Delay2/1, Gateway Out4/1
  en/1 -> Gateway Out3/1, Logical5/2
  Delay2/1 -> Logical1/2, tags_received/1, Gateway Out6/1, Gateway Out12/1
  Constant1/1 -> Relational/2
  load/1 -> Gateway Out9/1, Gateway Out8/1, quadrant_offset_count/1, Logical12/1, Gateway Out/1
  quadrant_offset_count/1 -> Gateway Out11/1, quadrant_offset/1
  tag/1 -> Gateway Out2/1, Relational/1
  Relational/1 -> Logical5/1
  Logical1/1 -> Gateway Out10/1, quadrant_offset_count/2, Gateway Out13/1, Gateway Out7/1, Logical12/2
  Logical12/1 -> Delay2/2, Gateway Out5/1
  previous_quadrant/1 -> Gateway Out14/1, edge_detect/1, Gateway Out1/1
  Gateway Out2/1 -> Scope/3
  Gateway Out3/1 -> Scope/4
  Gateway Out1/1 -> Scope/2
  Gateway Out/1 -> Scope/1
  Gateway Out4/1 -> Scope/5
  Gateway Out5/1 -> Scope/6
  Gateway Out6/1 -> Scope/7
  Gateway Out7/1 -> Scope/8
  Gateway Out8/1 -> Scope1/1
  Gateway Out9/1 -> Scope1/2
  Gateway Out10/1 -> Scope1/3
  Gateway Out11/1 -> Scope1/4
  Gateway Out13/1 -> Scope2/4
  Gateway Out12/1 -> Scope2/3
  Gateway Out15/1 -> Scope2/2
  Gateway Out14/1 -> Scope2/1
  edge_detect/1 -> Logical1/1, Gateway Out15/1
